simulink model "UsefulModelForGraphics"  (R2021a)
settings: Solver=VariableStepAuto  StartTime=0.0  StopTime=10.0  RelTol=1e-3
values from neighbouring files (symbols this model uses):
  desideredSpeeds = 0:speedStep:maxSpeed    [identificateUSV.m]
  desideredYawRates = minYawRate:yawRateStep:maxYawRate    [identificateUSV.m]
  FFspeedCommands = interp1([0 speedMeanLevelSteps maxSpeed],                           [0 speedCommandLevelSteps 100],                            desideredSpeeds, 'pchip')    [identificateUSV.m]
  FFyawRateCommands = interp1([0 yawRateMeanLevelStepsFixed minYawRate maxYawRate],                              [0 yawRateCommandLevelStepsFixed -100 100],                              desideredYawRates, 'pchip')    [identificateUSV.m]
  lateralP1D = procest(idData,'P1D')    [identificateUSV.m]
  longitudinalP1D = procest(idData,'P1D')    [identificateUSV.m]
settings Model: Creator=frank  LastModifiedBy=frank

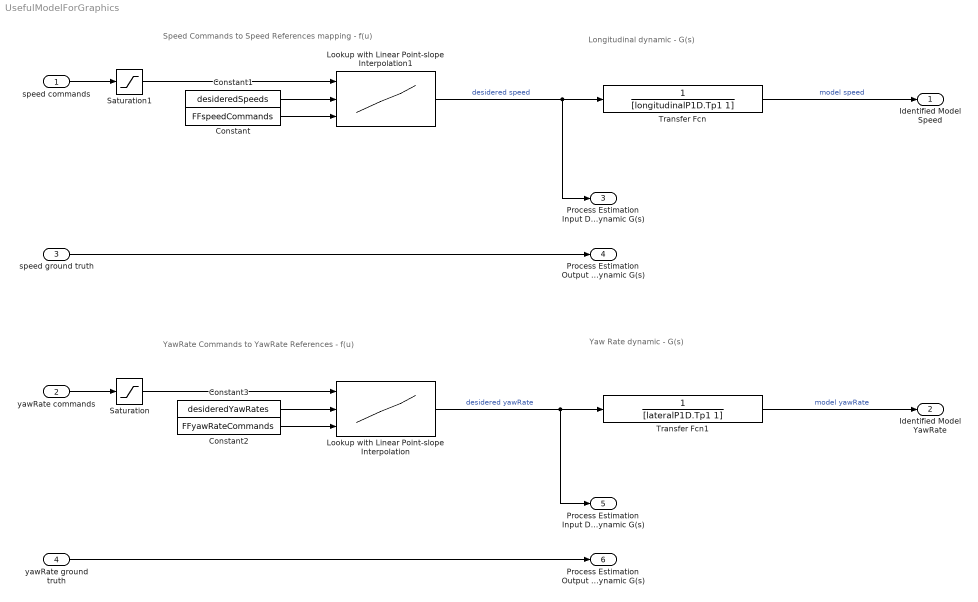
== system UsefulModelForGraphics ==
  note: Longitudinal dynamic - G(s)
  note: Speed Commands to Speed References mapping - f(u)
  note: YawRate Commands to YawRate References - f(u)
  note: Yaw Rate dynamic - G(s)
  speed commands : Inport
  yawRate commands : Inport  Port=2
  speed ground truth : Inport  Port=3
  yawRate ground truth : Inport  Port=4
  Constant : Constant  Value=FFspeedCommands
  Constant1 : Constant  Value=desideredSpeeds
  Constant2 : Constant  Value=FFyawRateCommands
  Constant3 : Constant  Value=desideredYawRates
  Lookup with Linear Point-slope Interpolation : Lookup_n-D  NumberOfTableDimensions=1  BreakpointsForDimension1Source=Input port  BreakpointsForDimension1=[-5:5]  TableSource=Input port  Table=tanh([-5:5])  InternalRulePriority=Speed  RndMeth=Simplest  InputSameDT=on
      settings: InputPortMap=u0,p221,p5
  Lookup with Linear Point-slope Interpolation1 : Lookup_n-D  NumberOfTableDimensions=1  BreakpointsForDimension1Source=Input port  BreakpointsForDimension1=[-5:5]  TableSource=Input port  Table=tanh([-5:5])  InternalRulePriority=Speed  RndMeth=Simplest  InputSameDT=on
      settings: InputPortMap=u0,p221,p5
  Saturation : Saturate  UpperLimit=60  LowerLimit=-60
  Saturation1 : Saturate  UpperLimit=80  LowerLimit=0
  Transfer Fcn : TransferFcn  Denominator=[longitudinalP1D.Tp1 1]
  Transfer Fcn1 : TransferFcn  Denominator=[lateralP1D.Tp1 1]
  Identified Model Speed : Outport
  Identified Model YawRate : Outport  Port=2
  Process Estimation Input Data for Longitudinal Dynamic G(s) : Outport  Port=3
  Process Estimation Output Data for Longitudinal Dynamic G(s) : Outport  Port=4
  Process Estimation Input Data for YawRate Dynamic G(s) : Outport  Port=5
  Process Estimation Output Data for YawRate Dynamic G(s) : Outport  Port=6
  wires:
  yawRate commands/1 -> Saturation/1
  Saturation1/1 -> Lookup with Linear Point-slope Interpolation1/1
  Transfer Fcn1/1 -> Identified Model YawRate/1  "model yawRate"
  Constant3/1 -> Lookup with Linear Point-slope Interpolation/2
  Constant/1 -> Lookup with Linear Point-slope Interpolation1/3
  speed commands/1 -> Saturation1/1
  Lookup with Linear Point-slope Interpolation1/1 -> Process Estimation Input Data for Longitudinal Dynamic G(s)/1, Transfer Fcn/1  "desidered speed"
  Transfer Fcn/1 -> Identified Model Speed/1  "model speed"
  Saturation/1 -> Lookup with Linear Point-slope Interpolation/1
  Constant2/1 -> Lookup with Linear Point-slope Interpolation/3
  Constant1/1 -> Lookup with Linear Point-slope Interpolation1/2
  Lookup with Linear Point-slope Interpolation/1 -> Process Estimation Input Data for YawRate Dynamic G(s)/1, Transfer Fcn1/1  "desidered yawRate"
  speed ground truth/1 -> Process Estimation Output Data for Longitudinal Dynamic G(s)/1
  yawRate ground truth/1 -> Process Estimation Output Data for YawRate Dynamic G(s)/1
